simulink model "test"  (R2021a)
settings: Solver=VariableStepAuto  StartTime=0.0  StopTime=10  RelTol=1e-3
settings Model: Creator=pierr  LastModifiedBy=pierr

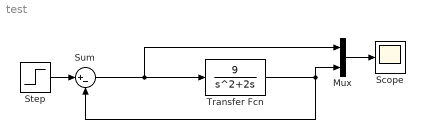
== system test ==
  Mux : Mux  Inputs=2
  Scope : Scope
  Step : Step  Time=0  SampleTime=0
  Sum : Sum  Inputs=|+-
  Transfer Fcn : TransferFcn  Numerator=[9]  Denominator=[1 2 0]
  wires:
  Sum/1 -> Mux/1, Transfer Fcn/1
  Transfer Fcn/1 -> Mux/2, Sum/2
  Step/1 -> Sum/1
  Mux/1 -> Scope/1
